simulink library "Energy_converter_Electrical_to_Mechanical"  (R2016a)
settings: Solver=ode1  StartTime=0.0  StopTime=Inf  FixedStep=0.001  RelTol=1e-3
undefined symbols (not defined in the file): API1dcac_efficiency, API2dcac_efficiency, API3dcac_efficiency, aux_power_state, AWR_InvStError, dat, DiscIntNeverNeededParam, EDCU_p_RefTqeMOT, emot_AcCmprFront_inertia, emot_AcCmprFront_nTab_3rdD, emot_AcCmprFront_pwrAC, emot_AcCmprFront_Tau, emot_AcCmprFront_trqTab_2ndD, emot_AcCmprFront_vltTab_1stD, emot_AcCmprRear_inertia, emot_AcCmprRear_nTab_3rdD, emot_AcCmprRear_pwrAC, emot_AcCmprRear_Tau, emot_AcCmprRear_trqTab_2ndD, emot_AcCmprRear_vltTab_1stD, emot_AirCmpr_inertia, emot_AirCmpr_nTab_3rdD, emot_AirCmpr_pwrAC, emot_AirCmpr_Tau, emot_AirCmpr_trqTab_2ndD, emot_AirCmpr_vltTab_1stD, emot_aircomp_power, emot_Cth_rotor, emot_Cth_stator, emot_dtrqEmotNeg, emot_dtrqEmotPtv, emot_inv_pwracTab_1st, emot_inv_pwrDC, emot_inv_pwrLoss, emot_inv_VrmsTab_2nd, emot_j, emot_mot_pwrLoss, emot_nTab_1stD, emot_pwrEtaTab_nRow, emot_pwrEtaTab_pwrTab, emot_pwrEtaTab_trqClm, emot_Rth_rotor_oil, emot_Rth_stator_oil, emot_Rth_stator_rotor, emot_tractiongroup, emot_Trotor_init, emot_trqMaxRow, emot_trqMinRow, emot_Tstator_init, emot_vltTab_3rdD, FirstDrivenAxleNoOfEmot, inv_Cth_cooling_plate, inv_Cth_diode, inv_Cth_IGBT, inv_n_IGBT_per_Switch, inv_Rth_cooling_plate_coolant, inv_Rth_PS_cooling_plate, inv_Tplate_init, inv_Tpowerstack_init, midAxleNoOfEmot ... (+6)
libraries: Electrical_converter x12, Energy_converter_Electrical_to_Mechanical x12, simulink x7
(part 2 of 8)

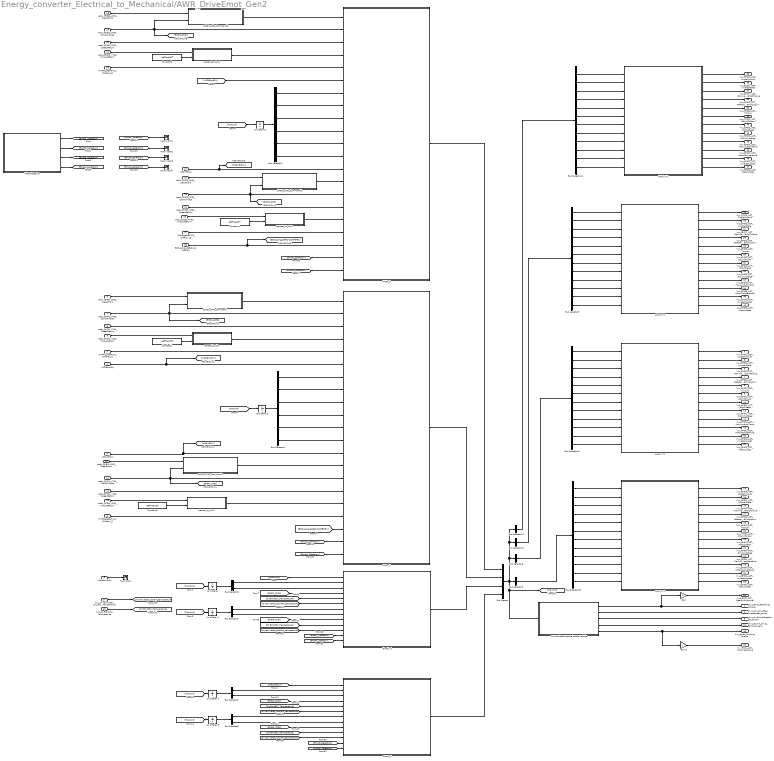
== system Energy_converter_Electrical_to_Mechanical/AWR_DriveEmot_Gen2 ==
  vltZkBmsPhy : Inport
  nGbxEM1In : Inport  Port=2
  ndotGbxEMIn : Inport  Port=3
  HVFreigabeHW1_SiRelay_D : Inport  Port=4
  HVFreigabeHW4_SiRelay_D : Inport  Port=5
  edcu_EMD1_CMD_ClearErrors : Inport  Port=6
  edcu_EMD1_CMD_ControlMode : Inport  Port=7
  edcu_EMD1_CMD_SpeedRefLim : Inport  Port=8
  edcu_EMD1_CMD_TorqueRefLim : Inport  Port=9
  edcu_EMD4_CMD_ClearErrors : Inport  Port=10
  edcu_EMD4_CMD_ControlMode : Inport  Port=11
  edcu_EMD4_CMD_SpeedRefLim : Inport  Port=12
  edcu_EMD4_CMD_TorqueRefLim : Inport  Port=13
  hvs_driveInverter_coolant_temperature : Inport  Port=14
  hvs_drvEmotOil_Temperature : Inport  Port=15
  HVFreigabeHW2_SiRelay_D : Inport  Port=16
  HVFreigabeHW3_SiRelay_D : Inport  Port=17
  edcu_EMD2_CMD_ClearErrors : Inport  Port=18
  edcu_EMD2_CMD_ControlMode : Inport  Port=19
  edcu_EMD2_CMD_SpeedRefLim : Inport  Port=20
  edcu_EMD2_CMD_TorqueRefLim : Inport  Port=21
  edcu_EMD3_CMD_ClearErrors : Inport  Port=22
  edcu_EMD3_CMD_ControlMode : Inport  Port=23
  edcu_EMD3_CMD_SpeedRefLim : Inport  Port=24
  edcu_EMD3_CMD_TorqueRefLim : Inport  Port=25
  EDCU_Dig_SafetyCutOffDG1 : Inport  Port=26
  nGbxEM2In : Inport  Port=27
  AWR 1 TX : Subsystem
  AWR 2 TX : Subsystem
  AWR 3 TX : Subsystem
  AWR 4 TX : Subsystem
  AWR1_4 : Subsystem
  AWR2_3 : Subsystem
  Bus Selector11 : BusSelector  OutputSignals=EMD2_ACT_DcLinkVoltage,EMD_ACT_DigitalInput1,EMD_ACT_MaximumAvailableTorque,EMD_ACT_DcLinkPower,EMD_ACT_MotorSpeed,EMD_ACT_MotorTorque,EMD_ACT_InverterState,EMD_ACT_ReferenceTorqueLimited,driveInverter_T_plate,drvEmot_T_Stator,Inv_Ploss,mot_Ploss
  Bus Selector14 : BusSelector  OutputSignals=EMD1_ACT_DcLinkVoltage,EMD_ACT_DigitalInput1,EMD_ACT_MaximumAvailableTorque,EMD_ACT_DcLinkPower,EMD_ACT_MotorSpeed,EMD_ACT_MotorTorque,EMD_ACT_InverterState,EMD_ACT_ReferenceTorqueLimited,driveInverter_T_plate,drvEmot_T_Stator,Inv_Ploss,mot_Ploss
  Bus Selector15 : BusSelector  OutputSignals=EMD4_ACT_DcLinkVoltage,EMD_ACT_DigitalInput1,EMD_ACT_MaximumAvailableTorque,EMD_ACT_DcLinkPower,EMD_ACT_MotorSpeed,EMD_ACT_MotorTorque,EMD_ACT_InverterState,EMD_ACT_ReferenceTorqueLimited,driveInverter_T_plate,drvEmot_T_Stator,Inv_Ploss,mot_Ploss
  Bus Selector9 : BusSelector  OutputSignals=EMD3_ACT_DcLinkVoltage,EMD_ACT_DigitalInput1,EMD_ACT_MaximumAvailableTorque,EMD_ACT_DcLinkPower,EMD_ACT_MotorSpeed,EMD_ACT_MotorTorque,EMD_ACT_InverterState,EMD_ACT_ReferenceTorqueLimited,driveInverter_T_plate,drvEmot_T_Stator,Inv_Ploss,mot_Ploss
  Bus Creator : BusCreator  Inputs=4
  Bus Selector1 : BusSelector  OutputSignals=awr1_4B.awr1B.EMD1_ACT_DcLinkVoltage,awr1_4B.awr1B.trqEmotDesPhy
  Bus Selector10 : BusSelector  OutputSignals=awr2_3B.awr3B.EMD3_ACT_DcLinkVoltage,awr2_3B.awr3B.EMD_ACT_DigitalInput1,awr2_3B.awr3B.EMD_ACT_MaximumAvailableTorque,awr2_3B.awr3B.EMD_ACT_DcLinkPower,awr2_3B.awr3B.EMD_ACT_MotorSpeed,awr2_3B.awr3B.EMD_ACT_MotorTorque,awr2_3B.awr3B.EMD_ACT_InverterState,awr2_3B.awr3B.EMD_ACT_ReferenceTorqueLimited,awr2_3B.awr3B.trqEmotDesPhy,emot2_3B.emot3B.driveInverter_T_plate,emot2_3B.emot3B.drvEmot_T_Stator,emot2_3B.emot3B.Inv_Ploss,emot2_3B.emot3B.mot_Ploss  OutputAsBus=on
  Bus Selector12 : BusSelector  OutputSignals=awr2_3B.awr2B.EMD2_ACT_DcLinkVoltage,awr2_3B.awr2B.EMD_ACT_DigitalInput1,awr2_3B.awr2B.EMD_ACT_MaximumAvailableTorque,awr2_3B.awr2B.EMD_ACT_DcLinkPower,awr2_3B.awr2B.EMD_ACT_MotorSpeed,awr2_3B.awr2B.EMD_ACT_MotorTorque,awr2_3B.awr2B.EMD_ACT_InverterState,awr2_3B.awr2B.EMD_ACT_ReferenceTorqueLimited,awr2_3B.awr2B.trqEmotDesPhy,emot2_3B.emot2B.driveInverter_T_plate,emot2_3B.emot2B.drvEmot_T_Stator,emot2_3B.emot2B.Inv_Ploss,emot2_3B.emot2B.mot_Ploss  OutputAsBus=on
  Bus Selector2 : BusSelector  OutputSignals=awr1_4B.awr4B.EMD4_ACT_DcLinkVoltage,awr1_4B.awr4B.trqEmotDesPhy
  Bus Selector3 : BusSelector  OutputSignals=emot2_3B.emot2B.trqEmotPhy,emot2_3B.emot3B.trqEmotPhy,emot2_3B.emot2B.pwrEmotPhy,emot2_3B.emot3B.pwrEmotPhy,emot2_3B.emot2B.trqEmotMax,emot2_3B.emot3B.trqEmotMax
  Bus Selector4 : BusSelector  OutputSignals=emot1_4B.emot1B.trqEmotPhy,emot1_4B.emot4B.trqEmotPhy,emot1_4B.emot1B.pwrEmotPhy,emot1_4B.emot4B.pwrEmotPhy,emot1_4B.emot1B.trqEmotMax,emot1_4B.emot4B.trqEmotMax
  Bus Selector5 : BusSelector  OutputSignals=awr1_4B.awr4B.EMD4_ACT_DcLinkVoltage,awr1_4B.awr4B.EMD_ACT_DigitalInput1,awr1_4B.awr4B.EMD_ACT_MaximumAvailableTorque,awr1_4B.awr4B.EMD_ACT_DcLinkPower,awr1_4B.awr4B.EMD_ACT_MotorSpeed,awr1_4B.awr4B.EMD_ACT_MotorTorque,awr1_4B.awr4B.EMD_ACT_InverterState,awr1_4B.awr4B.EMD_ACT_ReferenceTorqueLimited,awr1_4B.awr4B.trqEmotDesPhy,emot1_4B.emot4B.driveInverter_T_plate,emot1_4B.emot4B.drvEmot_T_Stator,emot1_4B.emot4B.Inv_Ploss,emot1_4B.emot4B.mot_Ploss  OutputAsBus=on
  Bus Selector6 : BusSelector  OutputSignals=awr1_4B.awr1B.EMD1_ACT_DcLinkVoltage,awr1_4B.awr1B.EMD_ACT_DigitalInput1,awr1_4B.awr1B.EMD_ACT_MaximumAvailableTorque,awr1_4B.awr1B.EMD_ACT_DcLinkPower,awr1_4B.awr1B.EMD_ACT_MotorSpeed,awr1_4B.awr1B.EMD_ACT_MotorTorque,awr1_4B.awr1B.EMD_ACT_InverterState,awr1_4B.awr1B.EMD_ACT_ReferenceTorqueLimited,awr1_4B.awr1B.trqEmotDesPhy,emot1_4B.emot1B.driveInverter_T_plate,emot1_4B.emot1B.drvEmot_T_Stator,emot1_4B.emot1B.Inv_Ploss,emot1_4B.emot1B.mot_Ploss  OutputAsBus=on
  Bus Selector7 : BusSelector  OutputSignals=awr2_3B.awr2B.EMD2_ACT_DcLinkVoltage,awr2_3B.awr2B.trqEmotDesPhy
  Bus Selector8 : BusSelector  OutputSignals=awr2_3B.awr3B.EMD3_ACT_DcLinkVoltage,awr2_3B.awr3B.trqEmotDesPhy
  Constant{1..4} (4 alike) : Constant  Value=RefTqeMOT
  EMD1_CMD_Command : Subsystem
  EMD1_CMD_Command1 : Subsystem
  EMD1_CMD_Command2 : Subsystem
  EMD1_CMD_Command3 : Subsystem
  Emot1_4 : Subsystem
  Emot2_3 : Subsystem
  Gain : Gain
  Gain1 : Gain
  MotorSelection : Subsystem
  SummarizeEmotorValuesForVehicle : Subsystem  TreatAsAtomicUnit=on
  Terminator{,1..4} (5 alike) : Terminator
  Unit Delay{,1..5} (6 alike) : UnitDelay  SampleTime=-1
  percent_to_Nm : Subsystem
  percent_to_Nm1 : Subsystem
  percent_to_Nm2 : Subsystem
  percent_to_Nm3 : Subsystem
  hvs_emot_RearAxle_torque : Outport
  hvs_driveInverter_wasteHeat_power : Outport  Port=2
  hvs_drvEmotWasteHeat_power : Outport  Port=3
  hvs_EMD1_ACT_DigitalInput1 : Outport  Port=4
  hvs_EMD1_ACT_InverterState : Outport  Port=5
  hvs_EMD1_ACT_MaxAvailableTorque : Outport  Port=6
  hvs_EMD1_ACT_ReferenceTorqueLim : Outport  Port=7
  hvs_EMD1_ACT_Torque : Outport  Port=8
  hvs_EMD1_ACT_DcLinkPower : Outport  Port=9
  hvs_EMD1_ACT_MotorSpeed : Outport  Port=10
  hvs_EMD1_ACT_DcLinkVoltage : Outport  Port=11
  hvs_EMD1_ACT_MaxJunctionTemp : Outport  Port=12
  hvs_EMD1_ACT_MotorTemperature : Outport  Port=13
  hvs_EMD4_ACT_DigitalInput1 : Outport  Port=14
  hvs_EMD4_ACT_InverterState : Outport  Port=15
  hvs_EMD4_ACT_MaxAvailableTorque : Outport  Port=16
  hvs_EMD4_ACT_ReferenceTorqueLim : Outport  Port=17
  hvs_EMD4_ACT_Torque : Outport  Port=18
  hvs_EMD4_ACT_DcLinkPower : Outport  Port=19
  hvs_EMD4_ACT_MotorSpeed : Outport  Port=20
  hvs_EMD4_ACT_DcLinkVoltage : Outport  Port=21
  hvs_EMD4_ACT_MaxJunctionTemperature : Outport  Port=22
  hvs_EMD4_ACT_MotorTemperature : Outport  Port=23
  hvs_dcLink_drive_emot_current : Outport  Port=24
  hvs_EMD3_ACT_DigitalInput1 : Outport  Port=25
  hvs_EMD3_ACT_InverterState : Outport  Port=26
  hvs_EMD3_ACT_MaxAvailableTorque : Outport  Port=27
  hvs_EMD3_ACT_ReferenceTorqueLim : Outport  Port=28
  hvs_EMD3_ACT_Torque : Outport  Port=29
  hvs_EMD3_ACT_DcLinkPower : Outport  Port=30
  hvs_EMD3_ACT_MotorSpeed : Outport  Port=31
  hvs_EMD3_ACT_DcLinkVoltage : Outport  Port=32
  hvs_EMD3_ACT_MaxJunctionTemp : Outport  Port=33
  hvs_EMD3_ACT_MotorTemperature : Outport  Port=34
  hvs_EMD2_ACT_DigitalInput1 : Outport  Port=35
  hvs_EMD2_ACT_InverterState : Outport  Port=36
  hvs_EMD2_ACT_MaxAvailableTorque : Outport  Port=37
  hvs_EMD2_ACT_ReferenceTorqueLim : Outport  Port=38
  hvs_EMD2_ACT_Torque : Outport  Port=39
  hvs_EMD2_ACT_DcLinkPower : Outport  Port=40
  hvs_EMD2_ACT_MotorSpeed : Outport  Port=41
  hvs_EMD2_ACT_DcLinkVoltage : Outport  Port=42
  hvs_EMD2_ACT_MaxJunctionTemp : Outport  Port=43
  hvs_EMD2_ACT_MotorTemperature : Outport  Port=44
  hvs_emot_MidAxle_torque : Outport  Port=45
  hvs_EMD2_ACT_InverterLosses : Outport  Port=46
  hvs_EMD2_ACT_MotorLosses : Outport  Port=47
  hvs_EMD3_ACT_InverterLosses : Outport  Port=48
  hvs_EMD3_ACT_MotorLosses : Outport  Port=49
  hvs_EMD1_ACT_InverterLosses : Outport  Port=50
  hvs_EMD1_ACT_MotorLosses : Outport  Port=51
  hvs_EMD4_ACT_InverterLosses : Outport  Port=52
  hvs_EMD4_ACT_MotorLosses : Outport  Port=53
  hvs_EMD_ACT_RearAxle_torque : Outport  Port=54
  hvs_EMD_ACT_MidAxle_torque : Outport  Port=55
  wires:
  [Emot3_Selection] -> Emot2_3/13(Emot3_Selection)
  [Emot2_Selection] -> Emot2_3/12(Emot2_Selection)
  [Emot4_Selection] -> Emot1_4/13(Emot4_Selection)
  [Emot1_Selection] -> Emot1_4/12(Emot1_Selection)
  [Emot4_Selection] -> AWR1_4/21(Emot4_Selection)
  [Emot1_Selection] -> AWR1_4/20(Emot1_Selection)
  [Emot3_Selection] -> AWR2_3/21(Emot3_Selection)
  [Emot2_Selection] -> AWR2_3/20(Emot2_Selection)
  [Emot4_Selection] -> Terminator4/1
  [Emot3_Selection] -> Terminator3/1
  [Emot2_Selection] -> Terminator2/1
  [Emot1_Selection] -> Terminator1/1
  MotorSelection/4(Emot4_Selection) -> [Emot4_Selection]
  MotorSelection/3(Emot3_Selection) -> [Emot3_Selection]
  MotorSelection/2(Emot2_Selection) -> [Emot2_Selection]
  MotorSelection/1(Emot1_Selection) -> [Emot1_Selection]
  Gain1/1 -> hvs_EMD_ACT_MidAxle_torque/1  "hvs_EMD_ACT_MidAxle_torque"
  Gain/1 -> hvs_EMD_ACT_RearAxle_torque/1  "hvs_EMD_ACT_RearAxle_torque"
  ndotGbxEMIn/1 -> Terminator/1
  Bus Selector5/1 -> Bus Selector15/1  "TransInt"
  edcu_EMD1_CMD_ControlMode/1 -> EMD1_CMD_Command/2(EMD1_CMD_MotorControlMode), [EMD1_CMD], AWR1_4/2(EMD1_CMD_MotorControlMode)
  edcu_EMD1_CMD_TorqueRefLim/1 -> percent_to_Nm/1(Percentage_Torque)
  Constant1/1 -> percent_to_Nm/2(Reference_Torque)
  edcu_EMD1_CMD_ClearErrors/1 -> EMD1_CMD_Command/1(EMD1_CMD_ClearErrors)
  vltZkBmsPhy/1 -> AWR1_4/6(vltZkBmsPhy), [vltZkBmsPhy]
  nGbxEM1In/1 -> [nGbxEMIn], AWR1_4/13(nGbxEMIn)
  edcu_EMD4_CMD_ControlMode/1 -> EMD1_CMD_Command1/2(EMD1_CMD_MotorControlMode), [EMD4_CMD], AWR1_4/15(EMD4_CMD_MotorControlMode)
  edcu_EMD4_CMD_TorqueRefLim/1 -> percent_to_Nm1/1(Percentage_Torque)
  Constant2/1 -> percent_to_Nm1/2(Reference_Torque)
  edcu_EMD4_CMD_ClearErrors/1 -> EMD1_CMD_Command1/1(EMD1_CMD_ClearErrors)
  Bus Selector14/8 -> AWR 1 TX/8(IN_EMD1_ACT_ReferenceTorqueLimited)  "<EMD_ACT_ReferenceTorqueLimited>"
  Bus Selector14/7 -> AWR 1 TX/7(IN_EMD1_ACT_InverterState)  "<EMD_ACT_InverterState>"
  Bus Selector14/6 -> AWR 1 TX/6(IN_EMD1_ACT_Torque)  "<EMD_ACT_MotorTorque>"
  Bus Selector14/5 -> AWR 1 TX/5(IN_EMD1_ACT_MotorSpeed)  "<EMD_ACT_MotorSpeed>"
  Bus Selector14/4 -> AWR 1 TX/4(IN_EMD1_ACT_DcLinkPower)  "<EMD_ACT_DcLinkPower>"
  Bus Selector14/3 -> AWR 1 TX/3(IN_EMD1_ACT_MaximumAvailableTorque)  "<EMD_ACT_MaximumAvailableTorque>"
  Bus Selector14/2 -> AWR 1 TX/2(IN_EMD1_ACT_DigitalInput1)  "<EMD_ACT_DigitalInput1>"
  Bus Selector14/1 -> AWR 1 TX/1(IN_EMD1_ACT_DcLinkVoltage)  "<EMD1_ACT_DcLinkVoltage>"
  Bus Creator/1 -> [TransInt], SummarizeEmotorValuesForVehicle/1(MultiBus_Emot_Inv_1_4), Bus Selector5/1, Bus Selector12/1, Bus Selector10/1, Bus Selector6/1  "TransInt"
  Bus Selector15/10 -> AWR 4 TX/10(IN_EMD4_ACT_MotorTemperature)  "<drvEmot_T_Stator>"
  Bus Selector15/9 -> AWR 4 TX/9(IN_EMD4_ACT_MaxJunctionTemperature)  "<driveInverter_T_plate>"
  Bus Selector15/8 -> AWR 4 TX/8(IN_EMD4_ACT_ReferenceTorqueLimited)  "<EMD_ACT_ReferenceTorqueLimited>"
  Bus Selector15/7 -> AWR 4 TX/7(IN_EMD4_ACT_InverterState)  "<EMD_ACT_InverterState>"
  Bus Selector15/5 -> AWR 4 TX/5(IN_EMD4_ACT_MotorSpeed)  "<EMD_ACT_MotorSpeed>"
  Bus Selector15/6 -> AWR 4 TX/6(IN_EMD4_ACT_Torque)  "<EMD_ACT_MotorTorque>"
  Bus Selector15/4 -> AWR 4 TX/4(IN_EMD4_ACT_DcLinkPower)  "<EMD_ACT_DcLinkPower>"
  Bus Selector15/3 -> AWR 4 TX/3(IN_EMD4_ACT_MaximumAvailableTorque)  "<EMD_ACT_MaximumAvailableTorque>"
  Bus Selector15/2 -> AWR 4 TX/2(IN_EMD4_ACT_DigitalInput1)  "<EMD_ACT_DigitalInput1>"
  Bus Selector15/1 -> AWR 4 TX/1(IN_EMD4_ACT_DcLinkVoltage)  "<EMD4_ACT_DcLinkVoltage>"
  Bus Selector6/1 -> Bus Selector14/1  "TransInt"
  SummarizeEmotorValuesForVehicle/1(hvs_emot_RearAxle_torque) -> Gain/1, hvs_emot_RearAxle_torque/1
  SummarizeEmotorValuesForVehicle/4(hvs_dcLink_drive_emot_current) -> hvs_dcLink_drive_emot_current/1
  AWR 1 TX/1(hvs_EMD1_ACT_DigitalInput1) -> hvs_EMD1_ACT_DigitalInput1/1
  AWR 1 TX/2(hvs_EMD1_ACT_InverterState) -> hvs_EMD1_ACT_InverterState/1
  AWR 1 TX/3(hvs_EMD1_ACT_MaxAvailableTorque) -> hvs_EMD1_ACT_MaxAvailableTorque/1
  AWR 1 TX/4(hvs_EMD1_ACT_ReferenceTorqueLim) -> hvs_EMD1_ACT_ReferenceTorqueLim/1
  AWR 1 TX/5(hvs_EMD1_ACT_Torque) -> hvs_EMD1_ACT_Torque/1
  AWR 1 TX/6(hvs_EMD1_ACT_DcLinkPower) -> hvs_EMD1_ACT_DcLinkPower/1
  AWR 1 TX/7(hvs_EMD1_ACT_MotorSpeed) -> hvs_EMD1_ACT_MotorSpeed/1
  AWR 1 TX/8(hvs_EMD1_ACT_DcLinkVoltage) -> hvs_EMD1_ACT_DcLinkVoltage/1
  AWR 1 TX/9(hvs_EMD1_ACT_MaxJunctionTemp) -> hvs_EMD1_ACT_MaxJunctionTemp/1
  AWR 1 TX/10(hvs_EMD1_ACT_MotorTemperature) -> hvs_EMD1_ACT_MotorTemperature/1
  AWR 4 TX/1(hvs_EMD4_ACT_DigitalInput1) -> hvs_EMD4_ACT_DigitalInput1/1
  AWR 4 TX/2(hvs_EMD4_ACT_InverterState) -> hvs_EMD4_ACT_InverterState/1
  AWR 4 TX/3(hvs_EMD4_ACT_MaxAvailableTorque) -> hvs_EMD4_ACT_MaxAvailableTorque/1
  AWR 4 TX/4(hvs_EMD4_ACT_ReferenceTorqueLim) -> hvs_EMD4_ACT_ReferenceTorqueLim/1
  AWR 4 TX/5(hvs_EMD4_ACT_Torque) -> hvs_EMD4_ACT_Torque/1
  AWR 4 TX/6(hvs_EMD4_ACT_DcLinkPower) -> hvs_EMD4_ACT_DcLinkPower/1
  AWR 4 TX/7(hvs_EMD4_ACT_MotorSpeed) -> hvs_EMD4_ACT_MotorSpeed/1
  AWR 4 TX/8(hvs_EMD4_ACT_DcLinkVoltage) -> hvs_EMD4_ACT_DcLinkVoltage/1
  AWR 4 TX/9(hvs_EMD4_ACT_MaxJunctionTemperature) -> hvs_EMD4_ACT_MaxJunctionTemperature/1
  AWR 4 TX/10(hvs_EMD4_ACT_MotorTemperature) -> hvs_EMD4_ACT_MotorTemperature/1
  SummarizeEmotorValuesForVehicle/3(hvs_drvEmotWasteHeat_power) -> hvs_drvEmotWasteHeat_power/1
  SummarizeEmotorValuesForVehicle/2(hvs_driveInverter_wasteHeat_power) -> hvs_driveInverter_wasteHeat_power/1
  [TransInt] -> Unit Delay/1
  Unit Delay/1 -> Bus Selector1/1
  [TransInt] -> Unit Delay1/1
  Unit Delay1/1 -> Bus Selector2/1
  hvs_driveInverter_coolant_temperature/1 -> [driveInverter_coolant_temperature]
  hvs_drvEmotOil_Temperature/1 -> [drvEmotOil_Temperature]
  [TransInt] -> Unit Delay3/1
  Unit Delay3/1 -> Bus Selector4/1
  EMD1_CMD_Command/1(Out_EMD1_CMD_Command) -> AWR1_4/1(EMD1_CMD_Commamd)
  edcu_EMD1_CMD_SpeedRefLim/1 -> AWR1_4/3(EMD1_CMD_SpeedRefLim)
  percent_to_Nm/1(Torque_Nm) -> AWR1_4/4(EMD1_CMD_TorqueRefLim)
  HVFreigabeHW1_SiRelay_D/1 -> AWR1_4/5(HVFreigabeHW_SiRelay_D)
  EMD1_CMD_Command1/1(Out_EMD1_CMD_Command) -> AWR1_4/14(EMD4_CMD_Commamd)
  edcu_EMD4_CMD_SpeedRefLim/1 -> AWR1_4/16(EMD4_CMD_SpeedRefLim)
  percent_to_Nm1/1(Torque_Nm) -> AWR1_4/17(EMD4_CMD_TorqueRefLim)
  HVFreigabeHW4_SiRelay_D/1 -> AWR1_4/18(HVFreigabeHW4_SiRelay_D)
  AWR1_4/1(awr1_4B) -> Bus Creator/2
  edcu_EMD2_CMD_ControlMode/1 -> [EMD2_CMD], EMD1_CMD_Command2/2(EMD1_CMD_MotorControlMode), AWR2_3/2(EMD2_CMD_MotorControlMode)
  edcu_EMD2_CMD_TorqueRefLim/1 -> percent_to_Nm2/1(Percentage_Torque)
  Constant3/1 -> percent_to_Nm2/2(Reference_Torque)
  edcu_EMD2_CMD_ClearErrors/1 -> EMD1_CMD_Command2/1(EMD1_CMD_ClearErrors)
  edcu_EMD3_CMD_ControlMode/1 -> EMD1_CMD_Command3/2(EMD1_CMD_MotorControlMode), AWR2_3/15(EMD3_CMD_MotorControlMode), [EMD3_CMD]
  edcu_EMD3_CMD_TorqueRefLim/1 -> percent_to_Nm3/1(Percentage_Torque)
  Constant4/1 -> percent_to_Nm3/2(Reference_Torque)
  edcu_EMD3_CMD_ClearErrors/1 -> EMD1_CMD_Command3/1(EMD1_CMD_ClearErrors)
  [TransInt] -> Unit Delay2/1
  Unit Delay2/1 -> Bus Selector3/1
  EMD1_CMD_Command2/1(Out_EMD1_CMD_Command) -> AWR2_3/1(EMD2_CMD_Commamd)
  edcu_EMD2_CMD_SpeedRefLim/1 -> AWR2_3/3(EMD2_CMD_SpeedRefLim)
  percent_to_Nm2/1(Torque_Nm) -> AWR2_3/4(EMD2_CMD_TorqueRefLim)
  HVFreigabeHW2_SiRelay_D/1 -> AWR2_3/5(HVFreigabeHW2_SiRelay_D)
  EMD1_CMD_Command3/1(Out_EMD1_CMD_Command) -> AWR2_3/14(EMD3_CMD_Commamd)
  edcu_EMD3_CMD_SpeedRefLim/1 -> AWR2_3/16(EMD3_CMD_SpeedRefLim)
  percent_to_Nm3/1(Torque_Nm) -> AWR2_3/17(EMD3_CMD_TorqueRefLim)
  HVFreigabeHW3_SiRelay_D/1 -> AWR2_3/18(HVFreigabeHW3_SiRelay_D)
  [vltZkBmsPhy] -> AWR2_3/6(vltZkBmsPhy)
  nGbxEM2In/1 -> [nGbxEM2In], AWR2_3/13(nGbxEMIn)
  [nGbxEMIn] -> Emot1_4/1(nGbxEMIn)
  Bus Selector1/1 -> Emot1_4/2(voltBatHV1)  "<EMD1_ACT_DcLinkVoltage>"
  Bus Selector1/2 -> Emot1_4/3(trqEmotDesPhy1)  "<trqEmotDesPhy>"
  [EMD1_CMD] -> Emot1_4/4(emot_CMD1)
  Bus Selector2/1 -> Emot1_4/7(voltBatHV4)  "<EMD4_ACT_DcLinkVoltage>"
  Bus Selector2/2 -> Emot1_4/8(trqEmotDesPhy4)  "<trqEmotDesPhy>"
  [EMD4_CMD] -> Emot1_4/9(emot_CMD4)
  Emot1_4/1(emot1_4B) -> Bus Creator/3
  AWR2_3/1(awr2_3B) -> Bus Creator/1
  [TransInt] -> Unit Delay4/1
  Unit Delay4/1 -> Bus Selector7/1
  [TransInt] -> Unit Delay5/1
  Unit Delay5/1 -> Bus Selector8/1
  [nGbxEM2In] -> Emot2_3/1(nGbxEMIn)
  Bus Selector7/1 -> Emot2_3/2(voltBatHV2)  "<EMD2_ACT_DcLinkVoltage>"
  Bus Selector7/2 -> Emot2_3/3(trqEmotDesPhy2)  "<trqEmotDesPhy>"
  [EMD2_CMD] -> Emot2_3/4(emot_CMD2)
  Bus Selector8/1 -> Emot2_3/7(voltBatHV3)  "<EMD3_ACT_DcLinkVoltage>"
  Bus Selector8/2 -> Emot2_3/8(trqEmotDesPhy3)  "<trqEmotDesPhy>"
  [EMD3_CMD] -> Emot2_3/9(emot_CMD3)
  Emot2_3/1(emot2_3B) -> Bus Creator/4
  Bus Selector9/10 -> AWR 3 TX/10(IN_EMD3_ACT_MotorTemperature)  "<drvEmot_T_Stator>"
  Bus Selector9/9 -> AWR 3 TX/9(IN_EMD3_ACT_MaxJunctionTemperature)  "<driveInverter_T_plate>"
  Bus Selector9/8 -> AWR 3 TX/8(IN_EMD3_ACT_ReferenceTorqueLimited)  "<EMD_ACT_ReferenceTorqueLimited>"
  Bus Selector9/7 -> AWR 3 TX/7(IN_EMD3_ACT_InverterState)  "<EMD_ACT_InverterState>"
  Bus Selector9/6 -> AWR 3 TX/6(IN_EMD3_ACT_Torque)  "<EMD_ACT_MotorTorque>"
  Bus Selector9/5 -> AWR 3 TX/5(IN_EMD3_ACT_MotorSpeed)  "<EMD_ACT_MotorSpeed>"
  Bus Selector9/4 -> AWR 3 TX/4(IN_EMD3_ACT_DcLinkPower)  "<EMD_ACT_DcLinkPower>"
  Bus Selector9/3 -> AWR 3 TX/3(IN_EMD3_ACT_MaximumAvailableTorque)  "<EMD_ACT_MaximumAvailableTorque>"
  Bus Selector9/2 -> AWR 3 TX/2(IN_EMD3_ACT_DigitalInput1)  "<EMD_ACT_DigitalInput1>"
  Bus Selector9/1 -> AWR 3 TX/1(IN_EMD3_ACT_DcLinkVoltage)  "<EMD3_ACT_DcLinkVoltage>"
  Bus Selector10/1 -> Bus Selector9/1  "TransInt"
  AWR 3 TX/1(hvs_EMD3_ACT_DigitalInput1) -> hvs_EMD3_ACT_DigitalInput1/1
  AWR 3 TX/2(hvs_EMD3_ACT_InverterState) -> hvs_EMD3_ACT_InverterState/1
  AWR 3 TX/3(hvs_EMD3_ACT_MaxAvailableTorque) -> hvs_EMD3_ACT_MaxAvailableTorque/1
  AWR 3 TX/4(hvs_EMD3_ACT_ReferenceTorqueLim) -> hvs_EMD3_ACT_ReferenceTorqueLim/1
  AWR 3 TX/5(hvs_EMD3_ACT_Torque) -> hvs_EMD3_ACT_Torque/1
  AWR 3 TX/6(hvs_EMD3_ACT_DcLinkPower) -> hvs_EMD3_ACT_DcLinkPower/1
  AWR 3 TX/7(hvs_EMD3_ACT_MotorSpeed) -> hvs_EMD3_ACT_MotorSpeed/1
  AWR 3 TX/8(hvs_EMD3_ACT_DcLinkVoltage) -> hvs_EMD3_ACT_DcLinkVoltage/1
  AWR 3 TX/9(hvs_EMD3_ACT_MaxJunctionTemp) -> hvs_EMD3_ACT_MaxJunctionTemp/1
  AWR 3 TX/10(hvs_EMD3_ACT_MotorTemperature) -> hvs_EMD3_ACT_MotorTemperature/1
  Bus Selector11/10 -> AWR 2 TX/10(IN_EMD2_ACT_MotorTemperature)  "<drvEmot_T_Stator>"
  Bus Selector11/9 -> AWR 2 TX/9(IN_EMD2_ACT_MaxJunctionTemperature)  "<driveInverter_T_plate>"
  Bus Selector11/8 -> AWR 2 TX/8(IN_EMD2_ACT_ReferenceTorqueLimited)  "<EMD_ACT_ReferenceTorqueLimited>"
  Bus Selector11/7 -> AWR 2 TX/7(IN_EMD2_ACT_InverterState)  "<EMD_ACT_InverterState>"
  Bus Selector11/6 -> AWR 2 TX/6(IN_EMD2_ACT_Torque)  "<EMD_ACT_MotorTorque>"
  Bus Selector11/5 -> AWR 2 TX/5(IN_EMD2_ACT_MotorSpeed)  "<EMD_ACT_MotorSpeed>"
  Bus Selector11/4 -> AWR 2 TX/4(IN_EMD2_ACT_DcLinkPower)  "<EMD_ACT_DcLinkPower>"
  Bus Selector11/3 -> AWR 2 TX/3(IN_EMD2_ACT_MaximumAvailableTorque)  "<EMD_ACT_MaximumAvailableTorque>"
  Bus Selector11/2 -> AWR 2 TX/2(IN_EMD2_ACT_DigitalInput1)  "<EMD_ACT_DigitalInput1>"
  Bus Selector11/1 -> AWR 2 TX/1(IN_EMD2_ACT_DcLinkVoltage)  "<EMD2_ACT_DcLinkVoltage>"
  Bus Selector12/1 -> Bus Selector11/1  "TransInt"
  AWR 2 TX/1(hvs_EMD2_ACT_DigitalInput1) -> hvs_EMD2_ACT_DigitalInput1/1
  AWR 2 TX/2(hvs_EMD2_ACT_InverterState) -> hvs_EMD2_ACT_InverterState/1
  AWR 2 TX/3(hvs_EMD2_ACT_MaxAvailableTorque) -> hvs_EMD2_ACT_MaxAvailableTorque/1
  AWR 2 TX/4(hvs_EMD2_ACT_ReferenceTorqueLim) -> hvs_EMD2_ACT_ReferenceTorqueLim/1
  AWR 2 TX/5(hvs_EMD2_ACT_Torque) -> hvs_EMD2_ACT_Torque/1
  AWR 2 TX/6(hvs_EMD2_ACT_DcLinkPower) -> hvs_EMD2_ACT_DcLinkPower/1
  AWR 2 TX/7(hvs_EMD2_ACT_MotorSpeed) -> hvs_EMD2_ACT_MotorSpeed/1
  AWR 2 TX/8(hvs_EMD2_ACT_DcLinkVoltage) -> hvs_EMD2_ACT_DcLinkVoltage/1
  AWR 2 TX/9(hvs_EMD2_ACT_MaxJunctionTemp) -> hvs_EMD2_ACT_MaxJunctionTemp/1
  AWR 2 TX/10(hvs_EMD2_ACT_MotorTemperature) -> hvs_EMD2_ACT_MotorTemperature/1
  EDCU_Dig_SafetyCutOffDG1/1 -> AWR2_3/19(EDCU_Dig_SafetyCutOffDG1), [EDCU_Dig_SafetyCutOffDG1]
  [EDCU_Dig_SafetyCutOffDG1] -> AWR1_4/19(EDCU_Dig_SafetyCutOffDG1)
  SummarizeEmotorValuesForVehicle/5(hvs_emot_MidAxle_torque) -> hvs_emot_MidAxle_torque/1, Gain1/1
  Bus Selector4/3 -> AWR1_4/9(pwEmot1Phy)  "<pwrEmotPhy>"
  Bus Selector4/4 -> AWR1_4/10(pwEmot4Phy)  "<pwrEmotPhy>"
  Bus Selector4/1 -> AWR1_4/7(trqEmot1Phy)  "<trqEmotPhy>"
  Bus Selector4/2 -> AWR1_4/8(trqEmot4Phy)  "<trqEmotPhy>"
  Bus Selector4/5 -> AWR1_4/11(trqEmot1Max)  "<trqEmotMax>"
  Bus Selector4/6 -> AWR1_4/12(trqEmot4Max)  "<trqEmotMax>"
  Bus Selector3/3 -> AWR2_3/9(pwEmot2Phy)  "<pwrEmotPhy>"
  Bus Selector3/4 -> AWR2_3/10(pwEmot3Phy)  "<pwrEmotPhy>"
  Bus Selector3/1 -> AWR2_3/7(trqEmot2Phy)  "<trqEmotPhy>"
  Bus Selector3/2 -> AWR2_3/8(trqEmot3Phy)  "<trqEmotPhy>"
  Bus Selector3/5 -> AWR2_3/11(trqEmot2Max)  "<trqEmotMax>"
  Bus Selector3/6 -> AWR2_3/12(trqEmot3Max)  "<trqEmotMax>"
  Bus Selector11/11 -> AWR 2 TX/11(IN_EMD2_ACT_InverterLosses)  "<Inv_Ploss>"
  Bus Selector11/12 -> AWR 2 TX/12(IN_EMD2_ACT_MotorLosses)  "<mot_Ploss>"
  Bus Selector14/11 -> AWR 1 TX/11(IN_EMD1_ACT_InverterLosses)  "<Inv_Ploss>"
  Bus Selector14/12 -> AWR 1 TX/12(IN_EMD1_ACT_MotorLosses)  "<mot_Ploss>"
  AWR 1 TX/11(hvs_EMD1_ACT_InverterLosses) -> hvs_EMD1_ACT_InverterLosses/1
  AWR 1 TX/12(hvs_EMD1_ACT_MotorLosses) -> hvs_EMD1_ACT_MotorLosses/1
  AWR 2 TX/11(hvs_EMD2_ACT_InverterLosses) -> hvs_EMD2_ACT_InverterLosses/1
  AWR 2 TX/12(hvs_EMD2_ACT_MotorLosses) -> hvs_EMD2_ACT_MotorLosses/1
  AWR 3 TX/11(hvs_EMD3_ACT_InverterLosses) -> hvs_EMD3_ACT_InverterLosses/1
  AWR 3 TX/12(hvs_EMD3_ACT_MotorLosses) -> hvs_EMD3_ACT_MotorLosses/1
  Bus Selector9/11 -> AWR 3 TX/11(IN_EMD3_ACT_InverterLosses)  "<Inv_Ploss>"
  Bus Selector9/12 -> AWR 3 TX/12(IN_EMD3_ACT_MotorLosses)  "<mot_Ploss>"
  AWR 4 TX/11(hvs_EMD4_ACT_InverterLosses) -> hvs_EMD4_ACT_InverterLosses/1
  AWR 4 TX/12(hvs_EMD4_ACT_MotorLosses) -> hvs_EMD4_ACT_MotorLosses/1
  Bus Selector15/11 -> AWR 4 TX/11(IN_EMD4_ACT_InverterLosses)  "<Inv_Ploss>"
  Bus Selector15/12 -> AWR 4 TX/12(IN_EMD4_ACT_MotorLosses)  "<mot_Ploss>"
  [driveInverter_coolant_temperature] -> Emot1_4/6(inv_coolant_temperature1)
  [drvEmotOil_Temperature] -> Emot1_4/5(emot_oil_temperature1)
  [drvEmotOil_Temperature] -> Emot1_4/10(emot_oil_temperature4)
  [driveInverter_coolant_temperature] -> Emot1_4/11(inv_coolant_temperature4)
  [drvEmotOil_Temperature] -> Emot2_3/5(emot_oil_temperature2)
  [driveInverter_coolant_temperature] -> Emot2_3/6(inv_coolant_temperature2)
  [drvEmotOil_Temperature] -> Emot2_3/10(emot_oil_temperature3)
  [driveInverter_coolant_temperature] -> Emot2_3/11(inv_coolant_temperature3)
  Bus Selector14/10 -> AWR 1 TX/10(IN_EMD1_ACT_MotorTemperature)  "<drvEmot_T_Stator>"
  Bus Selector14/9 -> AWR 1 TX/9(IN_EMD1_ACT_MaxJunctionTemperature)  "<driveInverter_T_plate>"

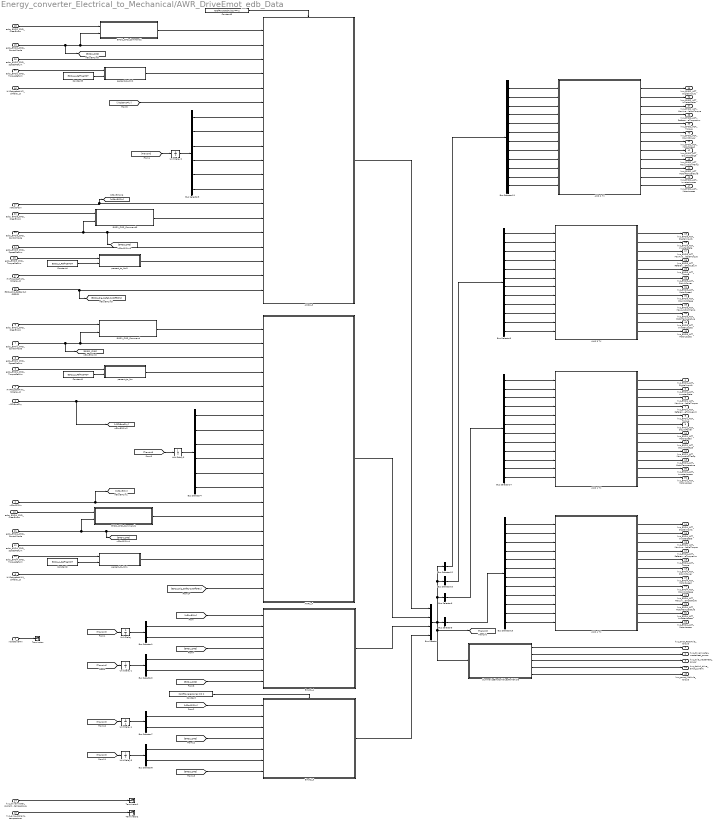
== system Energy_converter_Electrical_to_Mechanical/AWR_DriveEmot_edb_Data ==
  vltZkBmsPhy : Inport
  nGbxEM1In : Inport  Port=2
  ndotGbxEMIn : Inport  Port=3
  HVFreigabeHW1_SiRelay_D : Inport  Port=4
  HVFreigabeHW4_SiRelay_D : Inport  Port=5
  edcu_EMD1_CMD_ClearErrors : Inport  Port=6
  edcu_EMD1_CMD_ControlMode : Inport  Port=7
  edcu_EMD1_CMD_SpeedRefLim : Inport  Port=8
  edcu_EMD1_CMD_TorqueRefLim : Inport  Port=9
  edcu_EMD4_CMD_ClearErrors : Inport  Port=10
  edcu_EMD4_CMD_ControlMode : Inport  Port=11
  edcu_EMD4_CMD_SpeedRefLim : Inport  Port=12
  edcu_EMD4_CMD_TorqueRefLim : Inport  Port=13
  hvs_driveInverter_coolant_temperature : Inport  Port=14
  hvs_axle_coolant_temperature : Inport  Port=15
  HVFreigabeHW2_SiRelay_D : Inport  Port=16
  HVFreigabeHW3_SiRelay_D : Inport  Port=17
  edcu_EMD2_CMD_ClearErrors : Inport  Port=18
  edcu_EMD2_CMD_ControlMode : Inport  Port=19
  edcu_EMD2_CMD_SpeedRefLim : Inport  Port=20
  edcu_EMD2_CMD_TorqueRefLim : Inport  Port=21
  edcu_EMD3_CMD_ClearErrors : Inport  Port=22
  edcu_EMD3_CMD_ControlMode : Inport  Port=23
  edcu_EMD3_CMD_SpeedRefLim : Inport  Port=24
  edcu_EMD3_CMD_TorqueRefLim : Inport  Port=25
  EDCU_Dig_SafetyCutOffDG1 : Inport  Port=26
  nGbxEM2In : Inport  Port=27
  AWR 1 TX : Subsystem
  AWR 2 TX : Subsystem
  AWR 3 TX : Subsystem
  AWR 4 TX : Subsystem
  AWR1_4 : Subsystem
  AWR2_3 : Subsystem
  Bus Selector11 : BusSelector  OutputSignals=EMD2_ACT_DcLinkVoltage,EMD_ACT_DigitalInput1,EMD_ACT_MaximumAvailableTorque,EMD_ACT_DcLinkPower,EMD_ACT_MotorSpeed,EMD_ACT_MotorTorque,EMD_ACT_InverterState,EMD_ACT_ReferenceTorqueLimited,EMD_ACT_MaxJunctionTemperature,EMD_ACT_MotorTemperature,Inv_Ploss,mot_Ploss
  Bus Selector14 : BusSelector  OutputSignals=EMD1_ACT_DcLinkVoltage,EMD_ACT_DigitalInput1,EMD_ACT_MaximumAvailableTorque,EMD_ACT_DcLinkPower,EMD_ACT_MotorSpeed,EMD_ACT_MotorTorque,EMD_ACT_InverterState,EMD_ACT_ReferenceTorqueLimited,EMD_ACT_MaxJunctionTemperature,EMD_ACT_MotorTemperature,Inv_Ploss,mot_Ploss
  Bus Selector15 : BusSelector  OutputSignals=EMD4_ACT_DcLinkVoltage,EMD_ACT_DigitalInput1,EMD_ACT_MaximumAvailableTorque,EMD_ACT_DcLinkPower,EMD_ACT_MotorSpeed,EMD_ACT_MotorTorque,EMD_ACT_InverterState,EMD_ACT_ReferenceTorqueLimited,EMD_ACT_MaxJunctionTemperature,EMD_ACT_MotorTemperature,Inv_Ploss,mot_Ploss
  Bus Selector9 : BusSelector  OutputSignals=EMD3_ACT_DcLinkVoltage,EMD_ACT_DigitalInput1,EMD_ACT_MaximumAvailableTorque,EMD_ACT_DcLinkPower,EMD_ACT_MotorSpeed,EMD_ACT_MotorTorque,EMD_ACT_InverterState,EMD_ACT_ReferenceTorqueLimited,EMD_ACT_MaxJunctionTemperature,EMD_ACT_MotorTemperature,Inv_Ploss,mot_Ploss
  Bus Creator : BusCreator  Inputs=4
  Bus Selector1 : BusSelector  OutputSignals=awr1_4B.awr1B.EMD1_ACT_DcLinkVoltage,awr1_4B.awr1B.trqEmotDesPhy
  Bus Selector10 : BusSelector  OutputSignals=awr2_3B.awr3B.EMD3_ACT_DcLinkVoltage,awr2_3B.awr3B.EMD_ACT_DigitalInput1,awr2_3B.awr3B.EMD_ACT_MaximumAvailableTorque,awr2_3B.awr3B.EMD_ACT_DcLinkPower,awr2_3B.awr3B.EMD_ACT_MotorSpeed,awr2_3B.awr3B.EMD_ACT_MotorTorque,awr2_3B.awr3B.EMD_ACT_InverterState,awr2_3B.awr3B.EMD_ACT_ReferenceTorqueLimited,awr2_3B.awr3B.trqEmotDesPhy,awr2_3B.awr3B.EMD_ACT_MaxJunctionTemperature,awr2_3B.awr3B.EMD_ACT_MotorTemperature,emot2_3B.emot3B.Inv_Ploss,emot2_3B.emot3B.mot_Ploss  OutputAsBus=on
  Bus Selector12 : BusSelector  OutputSignals=awr2_3B.awr2B.EMD2_ACT_DcLinkVoltage,awr2_3B.awr2B.EMD_ACT_DigitalInput1,awr2_3B.awr2B.EMD_ACT_MaximumAvailableTorque,awr2_3B.awr2B.EMD_ACT_DcLinkPower,awr2_3B.awr2B.EMD_ACT_MotorSpeed,awr2_3B.awr2B.EMD_ACT_MotorTorque,awr2_3B.awr2B.EMD_ACT_InverterState,awr2_3B.awr2B.EMD_ACT_ReferenceTorqueLimited,awr2_3B.awr2B.trqEmotDesPhy,awr2_3B.awr2B.EMD_ACT_MaxJunctionTemperature,awr2_3B.awr2B.EMD_ACT_MotorTemperature,emot2_3B.emot2B.Inv_Ploss,emot2_3B.emot2B.mot_Ploss  OutputAsBus=on
  Bus Selector2 : BusSelector  OutputSignals=awr1_4B.awr4B.EMD4_ACT_DcLinkVoltage,awr1_4B.awr4B.trqEmotDesPhy
  Bus Selector3 : BusSelector  OutputSignals=emot2_3B.emot2B.trqEmotPhy,emot2_3B.emot3B.trqEmotPhy,emot2_3B.emot2B.pwrEmotPhy,emot2_3B.emot3B.pwrEmotPhy,emot2_3B.emot2B.trqEmotMax,emot2_3B.emot3B.trqEmotMax
  Bus Selector4 : BusSelector  OutputSignals=emot1_4B.emot1B.trqEmotPhy,emot1_4B.emot4B.trqEmotPhy,emot1_4B.emot1B.pwrEmotPhy,emot1_4B.emot4B.pwrEmotPhy,emot1_4B.emot1B.trqEmotMax,emot1_4B.emot4B.trqEmotMax
  Bus Selector5 : BusSelector  OutputSignals=awr1_4B.awr4B.EMD4_ACT_DcLinkVoltage,awr1_4B.awr4B.EMD_ACT_DigitalInput1,awr1_4B.awr4B.EMD_ACT_MaximumAvailableTorque,awr1_4B.awr4B.EMD_ACT_DcLinkPower,awr1_4B.awr4B.EMD_ACT_MotorSpeed,awr1_4B.awr4B.EMD_ACT_MotorTorque,awr1_4B.awr4B.EMD_ACT_InverterState,awr1_4B.awr4B.EMD_ACT_ReferenceTorqueLimited,awr1_4B.awr4B.trqEmotDesPhy,awr1_4B.awr4B.EMD_ACT_MaxJunctionTemperature,awr1_4B.awr4B.EMD_ACT_MotorTemperature,emot1_4B.emot4B.Inv_Ploss,emot1_4B.emot4B.mot_Ploss  OutputAsBus=on
  Bus Selector6 : BusSelector  OutputSignals=awr1_4B.awr1B.EMD1_ACT_DcLinkVoltage,awr1_4B.awr1B.EMD_ACT_DigitalInput1,awr1_4B.awr1B.EMD_ACT_MaximumAvailableTorque,awr1_4B.awr1B.EMD_ACT_DcLinkPower,awr1_4B.awr1B.EMD_ACT_MotorSpeed,awr1_4B.awr1B.EMD_ACT_MotorTorque,awr1_4B.awr1B.EMD_ACT_InverterState,awr1_4B.awr1B.EMD_ACT_ReferenceTorqueLimited,awr1_4B.awr1B.trqEmotDesPhy,awr1_4B.awr1B.EMD_ACT_MaxJunctionTemperature,awr1_4B.awr1B.EMD_ACT_MotorTemperature,emot1_4B.emot1B.Inv_Ploss,emot1_4B.emot1B.mot_Ploss  OutputAsBus=on
  Bus Selector7 : BusSelector  OutputSignals=awr2_3B.awr2B.EMD2_ACT_DcLinkVoltage,awr2_3B.awr2B.trqEmotDesPhy
  Bus Selector8 : BusSelector  OutputSignals=awr2_3B.awr3B.EMD3_ACT_DcLinkVoltage,awr2_3B.awr3B.trqEmotDesPhy
  Constant : Constant  Value=NoOfPoweredAxles == 2
  Constant{1..4} (4 alike) : Constant  Value=EDCU_p_RefTqeMOT
  Constant5 : Constant  Value=NoOfPoweredAxles == 2
  EMD1_CMD_Command : Subsystem
  EMD1_CMD_Command1 : Subsystem
  EMD1_CMD_Command2 : Subsystem
  EMD1_CMD_Command3 : Subsystem
  Emot1_4 : Subsystem
  Emot2_3 : Subsystem
  SummarizeEmotorValuesForVehicle : Subsystem  TreatAsAtomicUnit=on
  Terminator : Terminator
  Terminator1 : Terminator
  Terminator2 : Terminator
  Unit Delay{,1..5} (6 alike) : UnitDelay  SampleTime=-1
  percent_to_Nm : Subsystem
  percent_to_Nm1 : Subsystem
  percent_to_Nm2 : Subsystem
  percent_to_Nm3 : Subsystem
  hvs_emot_RearAxle_torque : Outport
  hvs_driveInverter_wasteHeat_power : Outport  Port=2
  hvs_axle_wasteHeat_power : Outport  Port=3
  hvs_EMD1_ACT_DigitalInput1 : Outport  Port=4
  hvs_EMD1_ACT_InverterState : Outport  Port=5
  hvs_EMD1_ACT_MaxAvailableTorque : Outport  Port=6
  hvs_EMD1_ACT_ReferenceTorqueLim : Outport  Port=7
  hvs_EMD1_ACT_Torque : Outport  Port=8
  hvs_EMD1_ACT_DcLinkPower : Outport  Port=9
  hvs_EMD1_ACT_MotorSpeed : Outport  Port=10
  hvs_EMD1_ACT_DcLinkVoltage : Outport  Port=11
  hvs_EMD1_ACT_MaxJunctionTemp : Outport  Port=12
  hvs_EMD1_ACT_MotorTemperature : Outport  Port=13
  hvs_EMD4_ACT_DigitalInput1 : Outport  Port=14
  hvs_EMD4_ACT_InverterState : Outport  Port=15
  hvs_EMD4_ACT_MaxAvailableTorque : Outport  Port=16
  hvs_EMD4_ACT_ReferenceTorqueLim : Outport  Port=17
  hvs_EMD4_ACT_Torque : Outport  Port=18
  hvs_EMD4_ACT_DcLinkPower : Outport  Port=19
  hvs_EMD4_ACT_MotorSpeed : Outport  Port=20
  hvs_EMD4_ACT_DcLinkVoltage : Outport  Port=21
  hvs_EMD4_ACT_MaxJunctionTemperature : Outport  Port=22
  hvs_EMD4_ACT_MotorTemperature : Outport  Port=23
  hvs_dcLink_drive_emot_current : Outport  Port=24
  hvs_EMD3_ACT_DigitalInput1 : Outport  Port=25
  hvs_EMD3_ACT_InverterState : Outport  Port=26
  hvs_EMD3_ACT_MaxAvailableTorque : Outport  Port=27
  hvs_EMD3_ACT_ReferenceTorqueLim : Outport  Port=28
  hvs_EMD3_ACT_Torque : Outport  Port=29
  hvs_EMD3_ACT_DcLinkPower : Outport  Port=30
  hvs_EMD3_ACT_MotorSpeed : Outport  Port=31
  hvs_EMD3_ACT_DcLinkVoltage : Outport  Port=32
  hvs_EMD3_ACT_MaxJunctionTemp : Outport  Port=33
  hvs_EMD3_ACT_MotorTemperature : Outport  Port=34
  hvs_EMD2_ACT_DigitalInput1 : Outport  Port=35
  hvs_EMD2_ACT_InverterState : Outport  Port=36
  hvs_EMD2_ACT_MaxAvailableTorque : Outport  Port=37
  hvs_EMD2_ACT_ReferenceTorqueLim : Outport  Port=38
  hvs_EMD2_ACT_Torque : Outport  Port=39
  hvs_EMD2_ACT_DcLinkPower : Outport  Port=40
  hvs_EMD2_ACT_MotorSpeed : Outport  Port=41
  hvs_EMD2_ACT_DcLinkVoltage : Outport  Port=42
  hvs_EMD2_ACT_MaxJunctionTemp : Outport  Port=43
  hvs_EMD2_ACT_MotorTemperature : Outport  Port=44
  hvs_emot_MidAxle_torque : Outport  Port=45
  hvs_EMD2_ACT_InverterLosses : Outport  Port=46
  hvs_EMD2_ACT_MotorLosses : Outport  Port=47
  hvs_EMD3_ACT_InverterLosses : Outport  Port=48
  hvs_EMD3_ACT_MotorLosses : Outport  Port=49
  hvs_EMD1_ACT_InverterLosses : Outport  Port=50
  hvs_EMD1_ACT_MotorLosses : Outport  Port=51
  hvs_EMD4_ACT_InverterLosses : Outport  Port=52
  hvs_EMD4_ACT_MotorLosses : Outport  Port=53
  wires:
  Constant5/1 -> AWR2_3/Enable
  Constant/1 -> Emot2_3/Enable
  ndotGbxEMIn/1 -> Terminator/1
  Bus Selector5/1 -> Bus Selector15/1  "TransInt"
  edcu_EMD1_CMD_ControlMode/1 -> [EMD1_CMD], EMD1_CMD_Command/2(EMD1_CMD_MotorControlMode), AWR1_4/2(EMD1_CMD_MotorControlMode)
  edcu_EMD1_CMD_TorqueRefLim/1 -> percent_to_Nm/1(Percentage_Torque)
  Constant1/1 -> percent_to_Nm/2(Reference_Torque)
  edcu_EMD1_CMD_ClearErrors/1 -> EMD1_CMD_Command/1(EMD1_CMD_ClearErrors)
  vltZkBmsPhy/1 -> [vltZkBmsPhy], AWR1_4/6(vltZkBmsPhy)
  nGbxEM1In/1 -> [nGbxEMIn], AWR1_4/13(nGbxEMIn)
  edcu_EMD4_CMD_ControlMode/1 -> EMD1_CMD_Command1/2(EMD1_CMD_MotorControlMode), [EMD4_CMD], AWR1_4/15(EMD4_CMD_MotorControlMode)
  edcu_EMD4_CMD_TorqueRefLim/1 -> percent_to_Nm1/1(Percentage_Torque)
  Constant2/1 -> percent_to_Nm1/2(Reference_Torque)
  edcu_EMD4_CMD_ClearErrors/1 -> EMD1_CMD_Command1/1(EMD1_CMD_ClearErrors)
  Bus Selector14/10 -> AWR 1 TX/10(IN_EMD1_ACT_MotorTemperature)  "<EMD_ACT_MotorTemperature>"
  Bus Selector14/9 -> AWR 1 TX/9(IN_EMD1_ACT_MaxJunctionTemperature)  "<EMD_ACT_MaxJunctionTemperature>"
  Bus Selector14/8 -> AWR 1 TX/8(IN_EMD1_ACT_ReferenceTorqueLimited)  "<EMD_ACT_ReferenceTorqueLimited>"
  Bus Selector14/7 -> AWR 1 TX/7(IN_EMD1_ACT_InverterState)  "<EMD_ACT_InverterState>"
  Bus Selector14/6 -> AWR 1 TX/6(IN_EMD1_ACT_Torque)  "<EMD_ACT_MotorTorque>"
  Bus Selector14/5 -> AWR 1 TX/5(IN_EMD1_ACT_MotorSpeed)  "<EMD_ACT_MotorSpeed>"
  Bus Selector14/4 -> AWR 1 TX/4(IN_EMD1_ACT_DcLinkPower)  "<EMD_ACT_DcLinkPower>"
  Bus Selector14/3 -> AWR 1 TX/3(IN_EMD1_ACT_MaximumAvailableTorque)  "<EMD_ACT_MaximumAvailableTorque>"
  Bus Selector14/2 -> AWR 1 TX/2(IN_EMD1_ACT_DigitalInput1)  "<EMD_ACT_DigitalInput1>"
  Bus Selector14/1 -> AWR 1 TX/1(IN_EMD1_ACT_DcLinkVoltage)  "<EMD1_ACT_DcLinkVoltage>"
  Bus Creator/1 -> [TransInt], SummarizeEmotorValuesForVehicle/1(MultiBus_Emot_Inv_1_4), Bus Selector5/1, Bus Selector12/1, Bus Selector10/1, Bus Selector6/1  "TransInt"
  Bus Selector15/10 -> AWR 4 TX/10(IN_EMD4_ACT_MotorTemperature)  "<EMD_ACT_MotorTemperature>"
  Bus Selector15/9 -> AWR 4 TX/9(IN_EMD4_ACT_MaxJunctionTemperature)  "<EMD_ACT_MaxJunctionTemperature>"
  Bus Selector15/8 -> AWR 4 TX/8(IN_EMD4_ACT_ReferenceTorqueLimited)  "<EMD_ACT_ReferenceTorqueLimited>"
  Bus Selector15/7 -> AWR 4 TX/7(IN_EMD4_ACT_InverterState)  "<EMD_ACT_InverterState>"
  Bus Selector15/5 -> AWR 4 TX/5(IN_EMD4_ACT_MotorSpeed)  "<EMD_ACT_MotorSpeed>"
  Bus Selector15/6 -> AWR 4 TX/6(IN_EMD4_ACT_Torque)  "<EMD_ACT_MotorTorque>"
  Bus Selector15/4 -> AWR 4 TX/4(IN_EMD4_ACT_DcLinkPower)  "<EMD_ACT_DcLinkPower>"
  Bus Selector15/3 -> AWR 4 TX/3(IN_EMD4_ACT_MaximumAvailableTorque)  "<EMD_ACT_MaximumAvailableTorque>"
  Bus Selector15/2 -> AWR 4 TX/2(IN_EMD4_ACT_DigitalInput1)  "<EMD_ACT_DigitalInput1>"
  Bus Selector15/1 -> AWR 4 TX/1(IN_EMD4_ACT_DcLinkVoltage)  "<EMD4_ACT_DcLinkVoltage>"
  Bus Selector6/1 -> Bus Selector14/1  "TransInt"
  SummarizeEmotorValuesForVehicle/1(hvs_emot_RearAxle_torque) -> hvs_emot_RearAxle_torque/1
  SummarizeEmotorValuesForVehicle/4(hvs_dcLink_drive_emot_current) -> hvs_dcLink_drive_emot_current/1
  AWR 1 TX/1(hvs_EMD1_ACT_DigitalInput1) -> hvs_EMD1_ACT_DigitalInput1/1
  AWR 1 TX/2(hvs_EMD1_ACT_InverterState) -> hvs_EMD1_ACT_InverterState/1
  AWR 1 TX/3(hvs_EMD1_ACT_MaxAvailableTorque) -> hvs_EMD1_ACT_MaxAvailableTorque/1
  AWR 1 TX/4(hvs_EMD1_ACT_ReferenceTorqueLim) -> hvs_EMD1_ACT_ReferenceTorqueLim/1
  AWR 1 TX/5(hvs_EMD1_ACT_Torque) -> hvs_EMD1_ACT_Torque/1
  AWR 1 TX/6(hvs_EMD1_ACT_DcLinkPower) -> hvs_EMD1_ACT_DcLinkPower/1
  AWR 1 TX/7(hvs_EMD1_ACT_MotorSpeed) -> hvs_EMD1_ACT_MotorSpeed/1
  AWR 1 TX/8(hvs_EMD1_ACT_DcLinkVoltage) -> hvs_EMD1_ACT_DcLinkVoltage/1
  AWR 1 TX/9(hvs_EMD1_ACT_MaxJunctionTemp) -> hvs_EMD1_ACT_MaxJunctionTemp/1
  AWR 1 TX/10(hvs_EMD1_ACT_MotorTemperature) -> hvs_EMD1_ACT_MotorTemperature/1
  AWR 4 TX/1(hvs_EMD4_ACT_DigitalInput1) -> hvs_EMD4_ACT_DigitalInput1/1
  AWR 4 TX/2(hvs_EMD4_ACT_InverterState) -> hvs_EMD4_ACT_InverterState/1
  AWR 4 TX/3(hvs_EMD4_ACT_MaxAvailableTorque) -> hvs_EMD4_ACT_MaxAvailableTorque/1
  AWR 4 TX/4(hvs_EMD4_ACT_ReferenceTorqueLim) -> hvs_EMD4_ACT_ReferenceTorqueLim/1
  AWR 4 TX/5(hvs_EMD4_ACT_Torque) -> hvs_EMD4_ACT_Torque/1
  AWR 4 TX/6(hvs_EMD4_ACT_DcLinkPower) -> hvs_EMD4_ACT_DcLinkPower/1
  AWR 4 TX/7(hvs_EMD4_ACT_MotorSpeed) -> hvs_EMD4_ACT_MotorSpeed/1
  AWR 4 TX/8(hvs_EMD4_ACT_DcLinkVoltage) -> hvs_EMD4_ACT_DcLinkVoltage/1
  AWR 4 TX/9(hvs_EMD4_ACT_MaxJunctionTemperature) -> hvs_EMD4_ACT_MaxJunctionTemperature/1
  AWR 4 TX/10(hvs_EMD4_ACT_MotorTemperature) -> hvs_EMD4_ACT_MotorTemperature/1
  SummarizeEmotorValuesForVehicle/3(hvs_axle_wasteHeat_power) -> hvs_axle_wasteHeat_power/1
  SummarizeEmotorValuesForVehicle/2(hvs_driveInverter_wasteHeat_power) -> hvs_driveInverter_wasteHeat_power/1
  [TransInt] -> Unit Delay/1
  Unit Delay/1 -> Bus Selector1/1
  [TransInt] -> Unit Delay1/1
  Unit Delay1/1 -> Bus Selector2/1
  hvs_driveInverter_coolant_temperature/1 -> Terminator1/1
  hvs_axle_coolant_temperature/1 -> Terminator2/1
  [TransInt] -> Unit Delay3/1
  Unit Delay3/1 -> Bus Selector4/1
  EMD1_CMD_Command/1(Out_EMD1_CMD_Command) -> AWR1_4/1(EMD1_CMD_Commamd)
  edcu_EMD1_CMD_SpeedRefLim/1 -> AWR1_4/3(EMD1_CMD_SpeedRefLim)
  percent_to_Nm/1(Torque_Nm) -> AWR1_4/4(EMD1_CMD_TorqueRefLim)
  HVFreigabeHW1_SiRelay_D/1 -> AWR1_4/5(HVFreigabeHW_SiRelay_D)
  EMD1_CMD_Command1/1(Out_EMD1_CMD_Command) -> AWR1_4/14(EMD4_CMD_Commamd)
  edcu_EMD4_CMD_SpeedRefLim/1 -> AWR1_4/16(EMD4_CMD_SpeedRefLim)
  percent_to_Nm1/1(Torque_Nm) -> AWR1_4/17(EMD4_CMD_TorqueRefLim)
  HVFreigabeHW4_SiRelay_D/1 -> AWR1_4/18(HVFreigabeHW4_SiRelay_D)
  AWR1_4/1(awr1_4B) -> Bus Creator/2
  edcu_EMD2_CMD_ControlMode/1 -> [EMD2_CMD], EMD1_CMD_Command2/2(EMD1_CMD_MotorControlMode), AWR2_3/2(EMD2_CMD_MotorControlMode)
  edcu_EMD2_CMD_TorqueRefLim/1 -> percent_to_Nm2/1(Percentage_Torque)
  Constant3/1 -> percent_to_Nm2/2(Reference_Torque)
  edcu_EMD2_CMD_ClearErrors/1 -> EMD1_CMD_Command2/1(EMD1_CMD_ClearErrors)
  edcu_EMD3_CMD_ControlMode/1 -> [EMD3_CMD], AWR2_3/15(EMD3_CMD_MotorControlMode), EMD1_CMD_Command3/2(EMD1_CMD_MotorControlMode)
  edcu_EMD3_CMD_TorqueRefLim/1 -> percent_to_Nm3/1(Percentage_Torque)
  Constant4/1 -> percent_to_Nm3/2(Reference_Torque)
  edcu_EMD3_CMD_ClearErrors/1 -> EMD1_CMD_Command3/1(EMD1_CMD_ClearErrors)
  [TransInt] -> Unit Delay2/1
  Unit Delay2/1 -> Bus Selector3/1
  EMD1_CMD_Command2/1(Out_EMD1_CMD_Command) -> AWR2_3/1(EMD2_CMD_Commamd)
  edcu_EMD2_CMD_SpeedRefLim/1 -> AWR2_3/3(EMD2_CMD_SpeedRefLim)
  percent_to_Nm2/1(Torque_Nm) -> AWR2_3/4(EMD2_CMD_TorqueRefLim)
  HVFreigabeHW2_SiRelay_D/1 -> AWR2_3/5(HVFreigabeHW2_SiRelay_D)
  EMD1_CMD_Command3/1(Out_EMD1_CMD_Command) -> AWR2_3/14(EMD3_CMD_Commamd)
  edcu_EMD3_CMD_SpeedRefLim/1 -> AWR2_3/16(EMD3_CMD_SpeedRefLim)
  percent_to_Nm3/1(Torque_Nm) -> AWR2_3/17(EMD3_CMD_TorqueRefLim)
  HVFreigabeHW3_SiRelay_D/1 -> AWR2_3/18(HVFreigabeHW3_SiRelay_D)
  [vltZkBmsPhy] -> AWR2_3/6(vltZkBmsPhy)
  nGbxEM2In/1 -> [nGbxEM2In], AWR2_3/13(nGbxEMIn)
  [nGbxEMIn] -> Emot1_4/1(nGbxEMIn)
  Bus Selector1/1 -> Emot1_4/2(voltBatHV1)  "<EMD1_ACT_DcLinkVoltage>"
  Bus Selector1/2 -> Emot1_4/3(trqEmotDesPhy1)  "<trqEmotDesPhy>"
  [EMD1_CMD] -> Emot1_4/4(emot_CMD1)
  Bus Selector2/1 -> Emot1_4/5(voltBatHV4)  "<EMD4_ACT_DcLinkVoltage>"
  Bus Selector2/2 -> Emot1_4/6(trqEmotDesPhy4)  "<trqEmotDesPhy>"
  [EMD4_CMD] -> Emot1_4/7(emot_CMD4)
  Emot1_4/1(emot1_4B) -> Bus Creator/3
  AWR2_3/1(awr2_3B) -> Bus Creator/1
  [TransInt] -> Unit Delay4/1
  Unit Delay4/1 -> Bus Selector7/1
  [TransInt] -> Unit Delay5/1
  Unit Delay5/1 -> Bus Selector8/1
  [nGbxEM2In] -> Emot2_3/1(nGbxEMIn)
  Bus Selector7/1 -> Emot2_3/2(voltBatHV2)  "<EMD2_ACT_DcLinkVoltage>"
  Bus Selector7/2 -> Emot2_3/3(trqEmotDesPhy2)  "<trqEmotDesPhy>"
  [EMD2_CMD] -> Emot2_3/4(emot_CMD2)
  Bus Selector8/1 -> Emot2_3/5(voltBatHV3)  "<EMD3_ACT_DcLinkVoltage>"
  Bus Selector8/2 -> Emot2_3/6(trqEmotDesPhy3)  "<trqEmotDesPhy>"
  [EMD3_CMD] -> Emot2_3/7(emot_CMD3)
  Emot2_3/1(emot2_3B) -> Bus Creator/4
  Bus Selector9/10 -> AWR 3 TX/10(IN_EMD3_ACT_MotorTemperature)  "<EMD_ACT_MotorTemperature>"
  Bus Selector9/9 -> AWR 3 TX/9(IN_EMD3_ACT_MaxJunctionTemperature)  "<EMD_ACT_MaxJunctionTemperature>"
  Bus Selector9/8 -> AWR 3 TX/8(IN_EMD3_ACT_ReferenceTorqueLimited)  "<EMD_ACT_ReferenceTorqueLimited>"
  Bus Selector9/7 -> AWR 3 TX/7(IN_EMD3_ACT_InverterState)  "<EMD_ACT_InverterState>"
  Bus Selector9/6 -> AWR 3 TX/6(IN_EMD3_ACT_Torque)  "<EMD_ACT_MotorTorque>"
  Bus Selector9/5 -> AWR 3 TX/5(IN_EMD3_ACT_MotorSpeed)  "<EMD_ACT_MotorSpeed>"
  Bus Selector9/4 -> AWR 3 TX/4(IN_EMD3_ACT_DcLinkPower)  "<EMD_ACT_DcLinkPower>"
  Bus Selector9/3 -> AWR 3 TX/3(IN_EMD3_ACT_MaximumAvailableTorque)  "<EMD_ACT_MaximumAvailableTorque>"
  Bus Selector9/2 -> AWR 3 TX/2(IN_EMD3_ACT_DigitalInput1)  "<EMD_ACT_DigitalInput1>"
  Bus Selector9/1 -> AWR 3 TX/1(IN_EMD3_ACT_DcLinkVoltage)  "<EMD3_ACT_DcLinkVoltage>"
  Bus Selector10/1 -> Bus Selector9/1  "TransInt"
  AWR 3 TX/1(hvs_EMD3_ACT_DigitalInput1) -> hvs_EMD3_ACT_DigitalInput1/1
  AWR 3 TX/2(hvs_EMD3_ACT_InverterState) -> hvs_EMD3_ACT_InverterState/1
  AWR 3 TX/3(hvs_EMD3_ACT_MaxAvailableTorque) -> hvs_EMD3_ACT_MaxAvailableTorque/1
  AWR 3 TX/4(hvs_EMD3_ACT_ReferenceTorqueLim) -> hvs_EMD3_ACT_ReferenceTorqueLim/1
  AWR 3 TX/5(hvs_EMD3_ACT_Torque) -> hvs_EMD3_ACT_Torque/1
  AWR 3 TX/6(hvs_EMD3_ACT_DcLinkPower) -> hvs_EMD3_ACT_DcLinkPower/1
  AWR 3 TX/7(hvs_EMD3_ACT_MotorSpeed) -> hvs_EMD3_ACT_MotorSpeed/1
  AWR 3 TX/8(hvs_EMD3_ACT_DcLinkVoltage) -> hvs_EMD3_ACT_DcLinkVoltage/1
  AWR 3 TX/9(hvs_EMD3_ACT_MaxJunctionTemp) -> hvs_EMD3_ACT_MaxJunctionTemp/1
  AWR 3 TX/10(hvs_EMD3_ACT_MotorTemperature) -> hvs_EMD3_ACT_MotorTemperature/1
  Bus Selector11/10 -> AWR 2 TX/10(IN_EMD2_ACT_MotorTemperature)  "<EMD_ACT_MotorTemperature>"
  Bus Selector11/9 -> AWR 2 TX/9(IN_EMD2_ACT_MaxJunctionTemperature)  "<EMD_ACT_MaxJunctionTemperature>"
  Bus Selector11/8 -> AWR 2 TX/8(IN_EMD2_ACT_ReferenceTorqueLimited)  "<EMD_ACT_ReferenceTorqueLimited>"
  Bus Selector11/7 -> AWR 2 TX/7(IN_EMD2_ACT_InverterState)  "<EMD_ACT_InverterState>"
  Bus Selector11/6 -> AWR 2 TX/6(IN_EMD2_ACT_Torque)  "<EMD_ACT_MotorTorque>"
  Bus Selector11/5 -> AWR 2 TX/5(IN_EMD2_ACT_MotorSpeed)  "<EMD_ACT_MotorSpeed>"
  Bus Selector11/4 -> AWR 2 TX/4(IN_EMD2_ACT_DcLinkPower)  "<EMD_ACT_DcLinkPower>"
  Bus Selector11/3 -> AWR 2 TX/3(IN_EMD2_ACT_MaximumAvailableTorque)  "<EMD_ACT_MaximumAvailableTorque>"
  Bus Selector11/2 -> AWR 2 TX/2(IN_EMD2_ACT_DigitalInput1)  "<EMD_ACT_DigitalInput1>"
  Bus Selector11/1 -> AWR 2 TX/1(IN_EMD2_ACT_DcLinkVoltage)  "<EMD2_ACT_DcLinkVoltage>"
  Bus Selector12/1 -> Bus Selector11/1  "TransInt"
  AWR 2 TX/1(hvs_EMD2_ACT_DigitalInput1) -> hvs_EMD2_ACT_DigitalInput1/1
  AWR 2 TX/2(hvs_EMD2_ACT_InverterState) -> hvs_EMD2_ACT_InverterState/1
  AWR 2 TX/3(hvs_EMD2_ACT_MaxAvailableTorque) -> hvs_EMD2_ACT_MaxAvailableTorque/1
  AWR 2 TX/4(hvs_EMD2_ACT_ReferenceTorqueLim) -> hvs_EMD2_ACT_ReferenceTorqueLim/1
  AWR 2 TX/5(hvs_EMD2_ACT_Torque) -> hvs_EMD2_ACT_Torque/1
  AWR 2 TX/6(hvs_EMD2_ACT_DcLinkPower) -> hvs_EMD2_ACT_DcLinkPower/1
  AWR 2 TX/7(hvs_EMD2_ACT_MotorSpeed) -> hvs_EMD2_ACT_MotorSpeed/1
  AWR 2 TX/8(hvs_EMD2_ACT_DcLinkVoltage) -> hvs_EMD2_ACT_DcLinkVoltage/1
  AWR 2 TX/9(hvs_EMD2_ACT_MaxJunctionTemp) -> hvs_EMD2_ACT_MaxJunctionTemp/1
  AWR 2 TX/10(hvs_EMD2_ACT_MotorTemperature) -> hvs_EMD2_ACT_MotorTemperature/1
  EDCU_Dig_SafetyCutOffDG1/1 -> [EDCU_Dig_SafetyCutOffDG1], AWR2_3/19(EDCU_Dig_SafetyCutOffDG1)
  [EDCU_Dig_SafetyCutOffDG1] -> AWR1_4/19(EDCU_Dig_SafetyCutOffDG1)
  SummarizeEmotorValuesForVehicle/5(hvs_emot_MidAxle_torque) -> hvs_emot_MidAxle_torque/1
  Bus Selector4/3 -> AWR1_4/9(pwEmot1Phy)  "<pwrEmotPhy>"
  Bus Selector4/4 -> AWR1_4/10(pwEmot4Phy)  "<pwrEmotPhy>"
  Bus Selector4/1 -> AWR1_4/7(trqEmot1Phy)  "<trqEmotPhy>"
  Bus Selector4/2 -> AWR1_4/8(trqEmot4Phy)  "<trqEmotPhy>"
  Bus Selector4/5 -> AWR1_4/11(trqEmot1Max)  "<trqEmotMax>"
  Bus Selector4/6 -> AWR1_4/12(trqEmot4Max)  "<trqEmotMax>"
  Bus Selector3/3 -> AWR2_3/9(pwEmot2Phy)  "<pwrEmotPhy>"
  Bus Selector3/4 -> AWR2_3/10(pwEmot3Phy)  "<pwrEmotPhy>"
  Bus Selector3/1 -> AWR2_3/7(trqEmot2Phy)  "<trqEmotPhy>"
  Bus Selector3/2 -> AWR2_3/8(trqEmot3Phy)  "<trqEmotPhy>"
  Bus Selector3/5 -> AWR2_3/11(trqEmot2Max)  "<trqEmotMax>"
  Bus Selector3/6 -> AWR2_3/12(trqEmot3Max)  "<trqEmotMax>"
  Bus Selector11/11 -> AWR 2 TX/11(IN_EMD2_ACT_InverterLosses)  "<Inv_Ploss>"
  Bus Selector11/12 -> AWR 2 TX/12(IN_EMD2_ACT_MotorLosses)  "<mot_Ploss>"
  Bus Selector14/11 -> AWR 1 TX/11(IN_EMD1_ACT_InverterLosses)  "<Inv_Ploss>"
  Bus Selector14/12 -> AWR 1 TX/12(IN_EMD1_ACT_MotorLosses)  "<mot_Ploss>"
  AWR 1 TX/11(hvs_EMD1_ACT_InverterLosses) -> hvs_EMD1_ACT_InverterLosses/1
  AWR 1 TX/12(hvs_EMD1_ACT_MotorLosses) -> hvs_EMD1_ACT_MotorLosses/1
  AWR 2 TX/11(hvs_EMD2_ACT_InverterLosses) -> hvs_EMD2_ACT_InverterLosses/1
  AWR 2 TX/12(hvs_EMD2_ACT_MotorLosses) -> hvs_EMD2_ACT_MotorLosses/1
  AWR 3 TX/11(hvs_EMD3_ACT_InverterLosses) -> hvs_EMD3_ACT_InverterLosses/1
  AWR 3 TX/12(hvs_EMD3_ACT_MotorLosses) -> hvs_EMD3_ACT_MotorLosses/1
  Bus Selector9/11 -> AWR 3 TX/11(IN_EMD3_ACT_InverterLosses)  "<Inv_Ploss>"
  Bus Selector9/12 -> AWR 3 TX/12(IN_EMD3_ACT_MotorLosses)  "<mot_Ploss>"
  AWR 4 TX/11(hvs_EMD4_ACT_InverterLosses) -> hvs_EMD4_ACT_InverterLosses/1
  AWR 4 TX/12(hvs_EMD4_ACT_MotorLosses) -> hvs_EMD4_ACT_MotorLosses/1
  Bus Selector15/11 -> AWR 4 TX/11(IN_EMD4_ACT_InverterLosses)  "<Inv_Ploss>"
  Bus Selector15/12 -> AWR 4 TX/12(IN_EMD4_ACT_MotorLosses)  "<mot_Ploss>"

== system Energy_converter_Electrical_to_Mechanical/Air Compressor ==
  hvs_inverterAirCompressor_coolant_temperature : Inport
  hvs_emot_AirCompressor_torque : Inport  Port=2
  Constant{,1..4} (5 alike) : Constant  Value=0
  Terminator : Terminator
  Terminator1 : Terminator
  "hvs_inverterAirCompressor_wasteHeat_power " : Outport
  hvs_emot_AirCompressor_angAcc : Outport  Port=2
  hvs_emot_AirCompressor_angPos : Outport  Port=3
  hvs_emot_AirCompressor_angVel : Outport  Port=4
  hvs_emot_AirCompressor_emot_current : Outport  Port=5
  wires:
  Constant/1 -> "hvs_inverterAirCompressor_wasteHeat_power "/1
  Constant1/1 -> hvs_emot_AirCompressor_angAcc/1
  Constant2/1 -> hvs_emot_AirCompressor_angPos/1
  Constant3/1 -> hvs_emot_AirCompressor_angVel/1
  Constant4/1 -> hvs_emot_AirCompressor_emot_current/1
  hvs_inverterAirCompressor_coolant_temperature/1 -> Terminator/1
  hvs_emot_AirCompressor_torque/1 -> Terminator1/1
